simulink model "Motorspeedcontrol"  (R2025b)
settings: Solver=VariableStepAuto  StartTime=0.0  StopTime=100.0  RelTol=1e-3
settings Model: Creator=ASUS  LastModifiedBy=ASUS

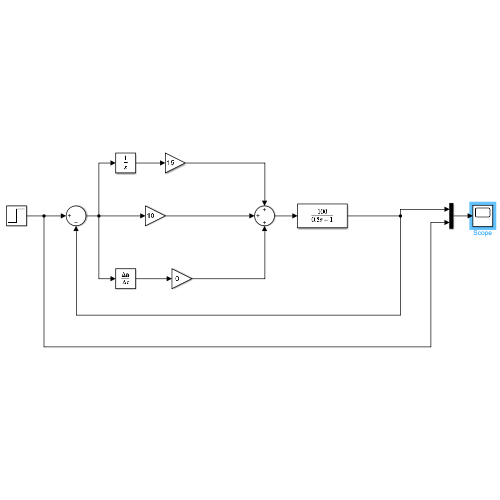
[thumbnail: Simulink's stored preview of the top-level diagram]
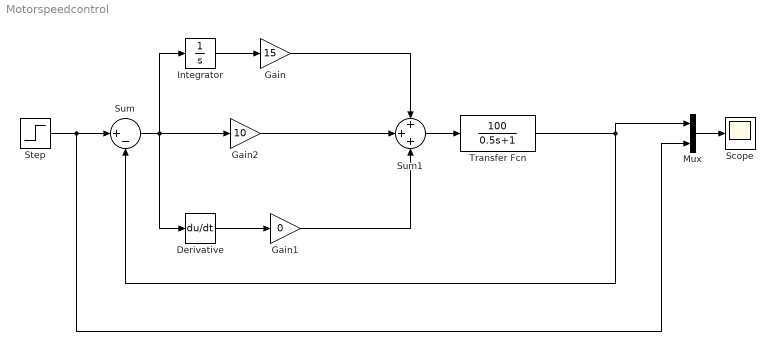
== system Motorspeedcontrol ==
  Derivative : Derivative
  Gain : Gain  Gain=15
  Gain1 : Gain  Gain=0
  Gain2 : Gain  Gain=10
  Integrator : Integrator
  Mux : Mux  Inputs=2
  Scope : Scope
      settings: ActiveDisplayYMinimum=96.769725505964672  ActiveDisplayYMaximum=101.04321533937004
  Step : Step  After=100  SampleTime=0
  Sum : Sum  Inputs=|+-
  Sum1 : Sum  Inputs=+++
  Transfer Fcn : TransferFcn  Numerator=[100]  Denominator=[0.5 1]
  wires:
  Transfer Fcn/1 -> Mux/1, Sum/2
  Sum/1 -> Derivative/1, Integrator/1, Gain2/1
  Gain2/1 -> Sum1/2
  Integrator/1 -> Gain/1
  Gain/1 -> Sum1/1
  Derivative/1 -> Gain1/1
  Gain1/1 -> Sum1/3
  Sum1/1 -> Transfer Fcn/1
  Step/1 -> Mux/2, Sum/1
  Mux/1 -> Scope/1
